simulink model "P1_Ex4"  (R2021a)
settings: Solver=FixedStepAuto  StartTime=0.0  StopTime=Total_time  RelTol=1e-3
PreLoadFcn:
  | PreLoad_P1_Ex4
StopFcn:
  | post_P1_Ex4
values from neighbouring files (symbols this model uses):
  Kt = 0.017    [PreLoad_P1_Ex4.m]
  Tg = 0.005    [PreLoad_P1_Ex4.m]
  Ts = 0.01    [PreLoad_P1_Ex4.m]
libraries: arduinolib x4, simulink x1
settings Model: SimulationMode=external  ExtModeTrigDuration=2  Creator=Eneko Lerma  LastModifiedBy=Control Automatic
settings SolverCC: AlgebraicLoopSolver=TrustRegion
settings DataIOCC: ReturnWorkspaceOutputs=off
settings OptimizationCC: EnhancedBackFolding=on  PassReuseOutputArgsAs=Individual arguments  MaxStackSize=64  OptimizeBlockOrder=speed  DifferentSizesBufferReuse=on  OptimizationCustomize=off  EfficientTunableParamExpr=on
settings DebuggingCC: ParameterPrecisionLossMsg=none  ParameterTunabilityLossMsg=error  SFMachineParentedDataDiag=warning  ArithmeticOperatorsInVariantConditions=warning
settings HardwareCC: ProdBitPerPointer=32  ProdBitPerSizeT=32  ProdBitPerPtrDiffT=32  ProdLargestAtomicInteger=Long  ProdLargestAtomicFloat=Double  ProdWordSize=32  ProdHWDeviceType=ARM Compatible->ARM Cortex
settings SFSimCC: SimUseLocalCustomCode=off  MATLABDynamicMemAlloc=off  CustomCodeUndefinedFunction=UseInterfaceOnly
settings RTWCC: SystemTargetFile=ert.tlc  HardwareBoard=Arduino Due  TemplateMakefile=ert_default_tmf  GenerateReport=on  RTWUseLocalCustomCode=off  Toolchain=Arduino ARM  BuildConfiguration=Faster Runs  IncludeHyperlinkInReport=on  LaunchReport=on  GenerateTraceInfo=on  GenerateTraceReport=on  GenerateTraceReportSl=on  GenerateTraceReportSf=on  GenerateTraceReportEml=on
settings RTWCC: CustomTerminator=|
  | writeDigitalPin((uint8_T)3, 0);
  | writeDigitalPin((uint8_T)5, 0);
settings CodeAppCC: ForceParamTrailComments=on  IgnoreCustomStorageClasses=off  OperatorAnnotations=on  SimulinkDataObjDesc=on  SFDataObjDesc=on  InsertBlockDesc=on
settings ERTTargetCC: SupportContinuousTime=on  SupportVariableSizeSignals=on

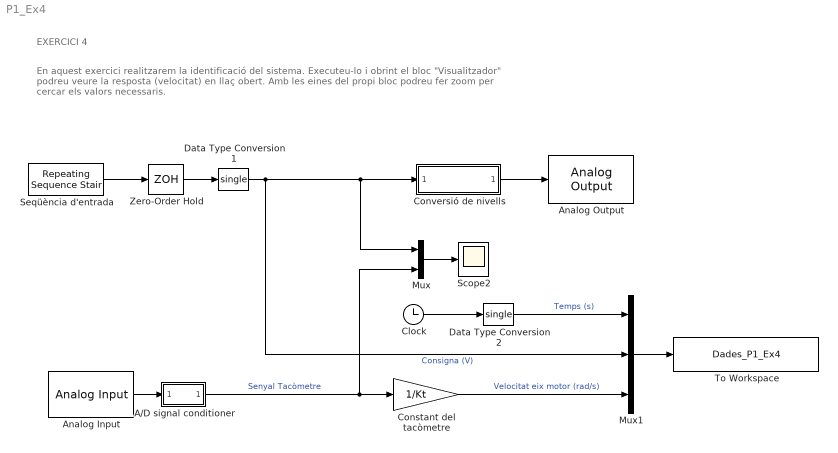
== system P1_Ex4 ==
  note: EXERCICI 4
  note: En aquest exercici realitzarem la identificació del sistema. Executeu-lo i obrint el bloc "Visualitzador"
      | podreu veure la resposta (velocitat) en llaç obert. Amb les eines del propi bloc podreu fer zoom per
      | cercar els valors necessaris.
  A/D signal conditioner : Subsystem
  Analog Input : arduinolib/Analog Input  pinNumber=0  ReadResultsOnly=off  ConversionTriggerSource=Software  ExternalTriggerType=uint32(0)  OutputDataType=uint16  EnableConversionCompleteNotify=off  EnableOuputStatus=off  SampleTime=Tg  blockPlatform=arduino
  Analog Output : arduinolib/Analog Output  DACpin=DAC1  blockPlatform=arduino
      settings: SourceProductBaseCode=ARDUINO
  Clock : Clock
  Constant del tacòmetre : Gain  Gain=1/Kt  OutDataTypeStr=single
  Conversió de nivells : Subsystem
  Data Type Conversion1 : DataTypeConversion  OutDataTypeStr=single
  Data Type Conversion2 : DataTypeConversion  OutDataTypeStr=single
  Mux : Mux  Inputs=2
  Mux1 : Mux  Inputs=3
  Scope2 : Scope
  Seqüència d'entrada : simulink/Sources/Repeating Sequence Stair  OutValues=input_vector  tsamp=t  OutMin=[]  OutMax=[]  OutDataTypeStr=float('double')  OutputDataTypeScalingMode=Specify via dialog  OutDataType=float('double')  ConRadixGroup=Best Precision: Vector-wise  OutScaling=2^-12
  To Workspace : ToWorkspace  VariableName=Dades_P1_Ex4  SampleTime=-1
  Zero-Order Hold : ZeroOrderHold  SampleTime=Ts
  wires:
  Mux/1 -> Scope2/1
  Conversió de nivells/1(" ") -> Analog Output/1
  Analog Input/1 -> A/D signal conditioner/1(" ")
  A/D signal conditioner/1(" ") -> Mux/2, Constant del tacòmetre/1  "Senyal Tacòmetre"
  Zero-Order Hold/1 -> Data Type Conversion1/1
  Clock/1 -> Data Type Conversion2/1
  Mux1/1 -> To Workspace/1
  Data Type Conversion1/1 -> Mux1/2, Conversió de nivells/1("  "), Mux/1  "Consigna (V)"
  Constant del tacòmetre/1 -> Mux1/3  "Velocitat eix motor (rad/s)"
  Seqüència d'entrada/1 -> Zero-Order Hold/1
  Data Type Conversion2/1 -> Mux1/1  "Temps (s)"

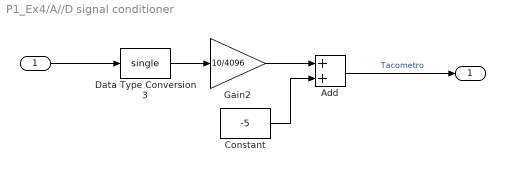
== system P1_Ex4/A//D signal conditioner ==
  " " : Inport
  Add : Sum  AccumDataTypeStr=single
  Constant : Constant  Value=-5  OutDataTypeStr=single
  Data Type Conversion3 : DataTypeConversion  OutDataTypeStr=single
  Gain2 : Gain  Gain=10/4096  OutDataTypeStr=single
  " " : Outport  VectorParamsAs1DForOutWhenUnconnected=off
  wires:
  " "/1 -> Data Type Conversion3/1
  Add/1 -> " "/1  "Tacometro"
  Gain2/1 -> Add/1
  Constant/1 -> Add/2
  Data Type Conversion3/1 -> Gain2/1

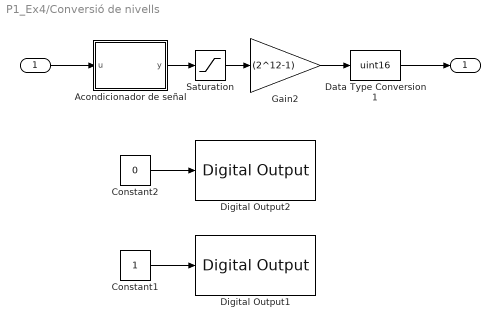
== system P1_Ex4/Conversió de nivells ==
  "  " : Inport  OutDataTypeStr=single
  Acondicionador de señal : MATLAB Function  TreatAsAtomicUnit=on
  Constant1 : Constant
  Constant2 : Constant  Value=0
  Data Type Conversion1 : DataTypeConversion  OutDataTypeStr=uint16
  Digital Output1 : arduinolib/Digital Output  pinNumber=5  Direction=output  blockPlatform=arduino
  Digital Output2 : arduinolib/Digital Output  pinNumber=3  Direction=output  blockPlatform=arduino
  Gain2 : Gain  Gain=(2^12-1)  OutDataTypeStr=single
  Saturation : Saturate  UpperLimit=1  LowerLimit=0  OutDataTypeStr=single
  " " : Outport  OutDataTypeStr=uint16  VectorParamsAs1DForOutWhenUnconnected=off
  wires:
  Saturation/1 -> Gain2/1
  Data Type Conversion1/1 -> " "/1
  Acondicionador de señal/1(y) -> Saturation/1
  "  "/1 -> Acondicionador de señal/1(u)
  Gain2/1 -> Data Type Conversion1/1
  Constant1/1 -> Digital Output1/1
  Constant2/1 -> Digital Output2/1

== matlab function P1_Ex4/Conversió de nivells/Acondicionador de señal ==
  data: u input; y output
function y = fcn(u)
y =0.0968*u+0.5058;
